simulink model "SiMappedEngine"  (R2023b)
settings: Solver=VariableStepAuto  StartTime=0.0  StopTime=inf  RelTol=1e-3  EnableMultiTasking=on
model workspace (MAT data in the model file):
  AccPwrTbl = Simulink.Parameter
  AccPwrTbl.Value = [0 0]
  AccPwrTbl.DataType = 'double'
  AccPwrTbl.Complexity = 'real'
  AccPwrTbl.Dimensions = [1 2]
  AccSpdBpts = Simulink.Parameter
  AccSpdBpts.Value = [300 750]
  AccSpdBpts.DataType = 'double'
  AccSpdBpts.Complexity = 'real'
  AccSpdBpts.Dimensions = [1 2]
  AfrStoich = Simulink.Parameter
  AfrStoich.Value = 14.6
  AfrStoich.DataType = 'double'
  AfrStoich.Complexity = 'real'
  AfrStoich.Dimensions = [1 1]
  Cps = Simulink.Parameter
  Cps.Value = 2
  Cps.DataType = 'double'
  Cps.Complexity = 'real'
  Cps.Dimensions = [1 1]
  NCyl = Simulink.Parameter
  NCyl.Value = 4
  NCyl.DataType = 'double'
  NCyl.Complexity = 'real'
  NCyl.Dimensions = [1 1]
  Pstd = Simulink.Parameter
  Pstd.Value = 101325
  Pstd.DataType = 'double'
  Pstd.Complexity = 'real'
  Pstd.Dimensions = [1 1]
  Rair = Simulink.Parameter
  Rair.Value = 287
  Rair.DataType = 'double'
  Rair.Complexity = 'real'
  Rair.Dimensions = [1 1]
  TimeCnstECP = Simulink.Parameter
  TimeCnstECP.Value = 0.125
  TimeCnstECP.DataType = 'double'
  TimeCnstECP.Complexity = 'real'
  TimeCnstECP.Dimensions = [1 1]
  TimeCnstEGR = Simulink.Parameter
  TimeCnstEGR.Value = 0.125
  TimeCnstEGR.DataType = 'double'
  TimeCnstEGR.Complexity = 'real'
  TimeCnstEGR.Dimensions = [1 1]
  TimeCnstETC = Simulink.Parameter
  TimeCnstETC.Value = 0.085
  TimeCnstETC.DataType = 'double'
  TimeCnstETC.Complexity = 'real'
  TimeCnstETC.Dimensions = [1 1]
  TimeCnstICP = Simulink.Parameter
  TimeCnstICP.Value = 0.125
  TimeCnstICP.DataType = 'double'
  TimeCnstICP.Complexity = 'real'
  TimeCnstICP.Dimensions = [1 1]
  TimeCnstIVL = Simulink.Parameter
  TimeCnstIVL.Value = 0.125
  TimeCnstIVL.DataType = 'double'
  TimeCnstIVL.Complexity = 'real'
  TimeCnstIVL.Dimensions = [1 1]
  TimeCnstMFA = Simulink.Parameter
  TimeCnstMFA.Value = 0.125
  TimeCnstMFA.DataType = 'double'
  TimeCnstMFA.Complexity = 'real'
  TimeCnstMFA.Dimensions = [1 1]
  TimeCnstSWVA = Simulink.Parameter
  TimeCnstSWVA.Value = 0.125
  TimeCnstSWVA.DataType = 'double'
  TimeCnstSWVA.Complexity = 'real'
  TimeCnstSWVA.Dimensions = [1 1]
  TimeCnstVCR = Simulink.Parameter
  TimeCnstVCR.Value = 0.125
  TimeCnstVCR.DataType = 'double'
  TimeCnstVCR.Complexity = 'real'
  TimeCnstVCR.Dimensions = [1 1]
  TimeCnstVGT = Simulink.Parameter
  TimeCnstVGT.Value = 0.15
  TimeCnstVGT.DataType = 'double'
  TimeCnstVGT.Complexity = 'real'
  TimeCnstVGT.Dimensions = [1 1]
  TimeCnstVIRL = Simulink.Parameter
  TimeCnstVIRL.Value = 0.125
  TimeCnstVIRL.DataType = 'double'
  TimeCnstVIRL.Complexity = 'real'
  TimeCnstVIRL.Dimensions = [1 1]
  TimeCnstWGA = Simulink.Parameter
  TimeCnstWGA.Value = 0.15
  TimeCnstWGA.DataType = 'double'
  TimeCnstWGA.Complexity = 'real'
  TimeCnstWGA.Dimensions = [1 1]
  Tstd = Simulink.Parameter
  Tstd.Value = 293.15
  Tstd.DataType = 'double'
  Tstd.Complexity = 'real'
  Tstd.Dimensions = [1 1]
  Vd = Simulink.Parameter
  Vd.Value = 0.0015
  Vd.DataType = 'double'
  Vd.Complexity = 'real'
  Vd.Dimensions = [1 1]
  f_air = Simulink.Parameter
  f_air.Value = [0 0 0 0 0 0 0 0 0 0 0 0 ... (256 elements, 16x16)]
  f_air.DataType = 'double'
  f_air.Complexity = 'real'
  f_air.Dimensions = [16 16]
  f_air_3d = Simulink.Parameter
  f_air_3d.Value = [0 0 0 0 0 0 0 0 0 0 0 0 ... (768 elements, 16x16x3)]
  f_air_3d.DataType = 'double'
  f_air_3d.Complexity = 'real'
  f_air_3d.Dimensions = [16 16 3]
  f_co = Simulink.Parameter
  f_co.Value = [0 0 0 0 0 0 0 0 0 0 0 0 ... (256 elements, 16x16)]
  f_co.DataType = 'double'
  f_co.Complexity = 'real'
  f_co.Dimensions = [16 16]
  f_co2 = Simulink.Parameter
  f_co2.Value = [0 0 0 0 0 0 0 0 0 0 0 0 ... (256 elements, 16x16)]
  f_co2.DataType = 'double'
  f_co2.Complexity = 'real'
  f_co2.Dimensions = [16 16]
  f_co2_3d = Simulink.Parameter
  f_co2_3d.Value = [0 0 0 0 0 0 0 0 0 0 0 0 ... (768 elements, 16x16x3)]
  f_co2_3d.DataType = 'double'
  f_co2_3d.Complexity = 'real'
  f_co2_3d.Dimensions = [16 16 3]
  f_co_3d = Simulink.Parameter
  f_co_3d.Value = [0 0 0 0 0 0 0 0 0 0 0 0 ... (768 elements, 16x16x3)]
  f_co_3d.DataType = 'double'
  f_co_3d.Complexity = 'real'
  f_co_3d.Dimensions = [16 16 3]
  f_eff = Simulink.Parameter
  f_eff.Value = [0 500 371.271960128 330.481212278 314.18997588 303.929242619 293.064446496 287.965450467 287.965450467 287.965450467 287.965450467 287.965450467 ... (256 elements, 16x16)]
  f_eff.DataType = 'double'
  f_eff.Complexity = 'real'
  f_eff.Dimensions = [16 16]
  f_eff_3d = Simulink.Parameter
  f_eff_3d.Value = [0 525 525 525 525 525 525 525 525 525 525 525 ... (768 elements, 16x16x3)]
  f_eff_3d.DataType = 'double'
  f_eff_3d.Complexity = 'real'
  f_eff_3d.Dimensions = [16 16 3]
  f_fuel = Simulink.Parameter
  f_fuel.Value = [0 0 0 0 0 0 0 0 0 0 0 0 ... (256 elements, 16x16)]
  f_fuel.DataType = 'double'
  f_fuel.Complexity = 'real'
  f_fuel.Dimensions = [16 16]
  f_fuel_3d = Simulink.Parameter
  f_fuel_3d.Value = [0 0 0 0 0 0 0 0 0 0 0 0 ... (768 elements, 16x16x3)]
  f_fuel_3d.DataType = 'double'
  f_fuel_3d.Complexity = 'real'
  f_fuel_3d.Dimensions = [16 16 3]
  f_hc = Simulink.Parameter
  f_hc.Value = [0 0 0 0 0 0 0 0 0 0 0 0 ... (256 elements, 16x16)]
  f_hc.DataType = 'double'
  f_hc.Complexity = 'real'
  f_hc.Dimensions = [16 16]
  f_hc_3d = Simulink.Parameter
  f_hc_3d.Value = [0 0 0 0 0 0 0 0 0 0 0 0 ... (768 elements, 16x16x3)]
  f_hc_3d.DataType = 'double'
  f_hc_3d.Complexity = 'real'
  f_hc_3d.Dimensions = [16 16 3]
  f_nox = Simulink.Parameter
  f_nox.Value = [0 0 0 0 0 0 0 0 0 0 0 0 ... (256 elements, 16x16)]
  f_nox.DataType = 'double'
  f_nox.Complexity = 'real'
  f_nox.Dimensions = [16 16]
  f_nox_3d = Simulink.Parameter
  f_nox_3d.Value = [0 0 0 0 0 0 0 0 0 0 0 0 ... (768 elements, 16x16x3)]
  f_nox_3d.DataType = 'double'
  f_nox_3d.Complexity = 'real'
  f_nox_3d.Dimensions = [16 16 3]
  f_pm = Simulink.Parameter
  f_pm.Value = [0  0  0  0  0  0  0  0  0  0  0  0  0  0  0  0; 0  0  0  0  0  0  0  0  0  0  0  0  0  0  0  0; 0  0  0  0  0  0  0  0  0  0  0  0  0  0  0  0; 0  0  0  0  0  0  0  0  0  0  0  0  0  0  0  0; 0  0  0  0  0  0  0  0  0  0  0  0  0  0  0  0; 0  0  0  0  0  0  0  0  0  0  0  0  0  0  0  0; 0  0  0  0  0  0  0  0  0  0  0  0  0  0  0  0; 0  0  0  0  0  0  0  0  0  0  0  0  0  0  0  0; 0  0  0  0  0  0  0  0  0  0  0  0  0  0  0  0; 0  0  0  0  0  0  0  0  0  0  0  0  0  0  0  0; 0  0  0  0  0  0  0  0  0  0  0  0  0  0  0  0; 0  0  0  0  0  0  0  0  0  0  0  0  0  0  0  0; 0  0  0  0  0  0  0  0  0  0  0  0  0  0  0  0; 0  0  0  0  0  0  0  0  0  0  0  0  0  0  0  0; 0  0  0  0  0  0  0  0  0  0  0  0  0  0  0  0; 0  0  0  0  0  0  0  0  0  0  0  0  0  0  0  0]
  f_pm.DataType = 'double'
  f_pm.Complexity = 'real'
  f_pm.Dimensions = [16 16]
  f_pm_3d = Simulink.Parameter
  f_pm_3d.Value = reshape([0 0 0 0 0 0 0 0 0 0 0 0 0 0 0 0 0 0 0 0 0 0 0 0 0 0 0 0 0 0 0 0 0 0 0 0 0 0 0 0 0 0 0 0 0 0 0 0 0 0 0 0 0 0 0 0 0 0 0 0 0 0 0 0 0 0 0 0 0 0 0 0 0 0 0 0 0 0 0 0 0 0 0 0 0 0 0 0 0 0 0 0 0 0 0 0 0 0 0 0 0 0 0 0 0 0 0 0 0 0 0 0 0 0 0 0 0 0 0 0 0 0 0 0 0 0 0 0 0 0 0 0 0 0 0 0 0 0 0 0 0 0 0 0 0 0 0 0 0 0 0 0 0 0 0 0 0 0 0 0 0 0 0 0 0 0 0 0 0 0 0 0 0 0 0 0 0 0 0 0 0 0 0 0 0 0 0 0 0 0 0 0 0 0 0 0 0 0 0 0 0 0 0 0 0 0 0 0 0 0 0 0 0 0 0 0 0 0 0 0 0 0 0 0 0 0 0 0 0 0 0 0 0 0 0 0 0 0 0 0 0 0 0 0 0 0 0 0 0 0 0 0 0 0 0 0 0 0 0 0 0 0 0 0 0 0 0 0 0 0 0 0 0 0 0 0 0 0 0 0 0 0 0 0 0 0 0 0 0 0 0 0 0 0 0 0 0 0 0 0 0 0 0 0 0 0 0 0 0 0 0 0 0 0 0 0 0 0 0 0 0 0 0 0 0 0 0 0 0 0 0 0 0 0 0 0 0 0 0 0 0 0 0 0 0 0 0 0 0 0 0 0 0 0 0 0 0 0 0 0 0 0 0 0 0 0 0 0 0 0 0 0 0 0 0 0 0 0 0 0 0 0 0 0 0 0 0 0 0 0 0 0 0 0 0 0 0 0 0 0 0 0 0 0 0 0 0 0 0 0 0 0 0 0 0 0 0 0 0 0 0 0 0 0 0 0 0 0 0 0 0 0 0 0 0 0 0 0 0 0 0 0 0 0 0 0 0 0 0 0 0 0 0 0 0 0 0 0 0 0 0 0 0 0 0 0 0 0 0 0 0 0 0 0 0 0 0 0 0 0 0 0 0 0 0 0 0 0 0 0 0 0 0 0 0 0 0 0 0 0 0 0 0 0 0 0 0 0 0 0 0 0 0 0 0 0 0 0 0 0 0 0 0 0 0 0 0 0 0 0 0 0 0 0 0 0 0 0 0 0 0 0 0 0 0 0 0 0 0 0 0 0 0 0 0 0 0 0 0 0 0 0 0 0 0 0 0 0 0 0 0 0 0 0 0 0 0 0 0 0 0 0 0 0 0 0 0 0 0 0 0 0 0 0 0 0 0 0 0 0 0 0 0 0 0 0 0 0 0 0 0 0 0 0 0 0 0 0 0 0 0 0 0 0 0 0 0 0 0 0 0 0 0 0 0 0 0 0 0 0 0 0 0 0 0 0 0 0 0 0 0 0 0 0 0 0 0 0 0 0 0 0 0 0 0 0 0 0 0 0 0 0 0 0 0 0 0 0 0 0 0 0 0 0 0 0 0 0 0 0 0 0 0 0 0 0 0 0 0 0 0 0 0 0 0 0 0 0 0 0 0 0 0 0 0 0 0 0 0 0 0 0 0 0 0 0 0 0 0 0 0 0 0 0 0 0 0 0 0 0 0 0 0 0 0 0 0 0 0 0 0 0 0 0 0 0 0 0 0 0 0 0 0 0 0 0 0 0], [16 16 3])
  f_pm_3d.DataType = 'double'
  f_pm_3d.Complexity = 'real'
  f_pm_3d.Dimensions = [16 16 3]
  f_tbrake = Simulink.Parameter
  f_tbrake.Value = [0 15 26.4285714286 37.8571428571 49.2857142857 60.7142857143 72.1428571429 75.6797764808 75.6797764808 75.6797764808 75.6797764808 75.6797764808 ... (256 elements, 16x16)]
  f_tbrake.DataType = 'double'
  f_tbrake.Complexity = 'real'
  f_tbrake.Dimensions = [16 16]
  f_tbrake_3d = Simulink.Parameter
  f_tbrake_3d.Value = [0 14.25 14.25 14.25 14.25 14.25 14.25 14.25 14.25 14.25 14.25 14.25 ... (768 elements, 16x16x3)]
  f_tbrake_3d.DataType = 'double'
  f_tbrake_3d.Complexity = 'real'
  f_tbrake_3d.Dimensions = [16 16 3]
  f_tbrake_engtmp_bpt = Simulink.Parameter
  f_tbrake_engtmp_bpt.Value = [233.15 273.15 373.15]
  f_tbrake_engtmp_bpt.DataType = 'double'
  f_tbrake_engtmp_bpt.Complexity = 'real'
  f_tbrake_engtmp_bpt.Dimensions = [1 3]
  f_tbrake_n_bpt = Simulink.Parameter
  f_tbrake_n_bpt.Value = [0 750 1053.57142857 1357.14285714 1660.71428571 1964.28571429 2267.85714286 2571.42857143 2875 3178.57142857 3482.14285714 3785.71428571 4089.28571429 4392.85714286 4696.42857143 5000]
  f_tbrake_n_bpt.DataType = 'double'
  f_tbrake_n_bpt.Complexity = 'real'
  f_tbrake_n_bpt.Dimensions = [1 16]
  f_tbrake_t_bpt = Simulink.Parameter
  f_tbrake_t_bpt.Value = [0 15 26.4285714286 37.8571428571 49.2857142857 60.7142857143 72.1428571429 83.5714285714 95 106.428571429 117.857142857 129.285714286 140.714285714 152.142857143 163.571428571 175]
  f_tbrake_t_bpt.DataType = 'double'
  f_tbrake_t_bpt.Complexity = 'real'
  f_tbrake_t_bpt.Dimensions = [1 16]
  f_texh = Simulink.Parameter
  f_texh.Value = [730.342454351 730.703124121 753.727232127 774.716518351 790.943395964 828.546144893 892.868946573 904.250339899 904.250339899 904.250339899 904.250339899 904.250339899 ... (256 elements, 16x16)]
  f_texh.DataType = 'double'
  f_texh.Complexity = 'real'
  f_texh.Dimensions = [16 16]
  f_texh_3d = Simulink.Parameter
  f_texh_3d.Value = [693.825331629 694.167967914 694.167967914 694.167967914 694.167967914 694.167967914 694.167967914 694.167967914 694.167967914 694.167967914 694.167967914 694.167967914 ... (768 elements, 16x16x3)]
  f_texh_3d.DataType = 'double'
  f_texh_3d.Complexity = 'real'
  f_texh_3d.Dimensions = [16 16 3]
  f_twc_eff_co = Simulink.Parameter
  f_twc_eff_co.Value = [0.17 0.25 0.45 0.99 0.99 0.99 0.99]
  f_twc_eff_co.DataType = 'double'
  f_twc_eff_co.Complexity = 'real'
  f_twc_eff_co.Dimensions = [1 7]
  f_twc_eff_hc = Simulink.Parameter
  f_twc_eff_hc.Value = [0.21 0.375 0.75 0.98 0.98 0.98 0.98]
  f_twc_eff_hc.DataType = 'double'
  f_twc_eff_hc.Complexity = 'real'
  f_twc_eff_hc.Dimensions = [1 7]
  f_twc_eff_lam = Simulink.Parameter
  f_twc_eff_lam.Value = [0.909090909 0.944055944 0.979020979 1 1.013986014 1.048951049 1.083916084]
  f_twc_eff_lam.DataType = 'double'
  f_twc_eff_lam.Complexity = 'real'
  f_twc_eff_lam.Dimensions = [1 7]
  f_twc_eff_nox = Simulink.Parameter
  f_twc_eff_nox.Value = [0.98 0.98 0.98 0.97 0.05 0.02 0]
  f_twc_eff_nox.DataType = 'double'
  f_twc_eff_nox.Complexity = 'real'
  f_twc_eff_nox.Dimensions = [1 7]
libraries: autolibhevctrlrcommon x1, autolibpowerinfoutils x1, autolibsharedmappedengines x1, autolibutils x1
(part 1 of 2)
settings Model: DataDictionary=SiMappedEngine.sldd  ModifiedByFormat=The MathWorks, Inc.  Creator=The MathWorks, Inc.  LastModifiedBy=The MathWorks, Inc.
settings SolverCC: AlgebraicLoopSolver=TrustRegion  DecoupledContinuousIntegration=on  MaxZcPerStep=1
settings DataIOCC: DSMLogging=off  ReturnWorkspaceOutputs=off
settings DebuggingCC: UnconnectedInputMsg=warning  UnconnectedOutputMsg=warning  UnconnectedLineMsg=warning  SubsystemReferenceDiagnosticForUnitTest=warning  ArithmeticOperatorsInVariantConditions=warning
settings ModelReferenceCC: EnableRefExpFcnMdlSchedulingChecks=on
settings SFSimCC: SimUseLocalCustomCode=off  CustomCodeUndefinedFunction=UseInterfaceOnly
settings RTWCC: RTWUseLocalCustomCode=off  DLArmComputeVersion=19.05
settings CodeAppCC: StateflowObjectComments=on
settings GRTTargetCC: TargetLangStandard=C89/C90 (ANSI)
settings ConfigComp: CovMetricSettings=dsw  CovSaveCumulativeToWorkspaceVar=on  CovSaveSingleToWorkspaceVar=on  CovExternalEMLEnable=off
settings SimscapeCC: SimscapeNormalizeSystem=off  SimscapeNominalValues={1, 'bar'; 1, 'cm^3/s'; 1, 'bar*kg/s'; 1, 'kJ/kg'; 1, 'kW'}

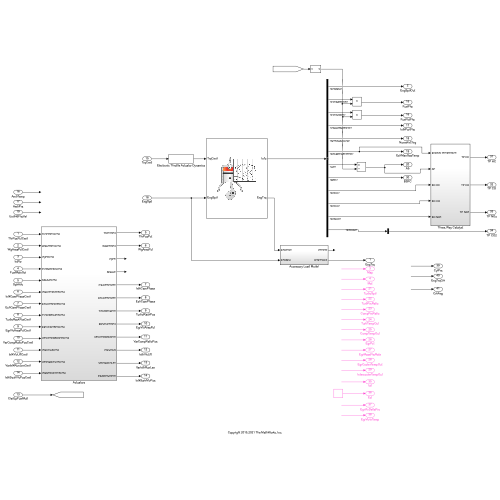
[thumbnail: Simulink's stored preview of the top-level diagram]
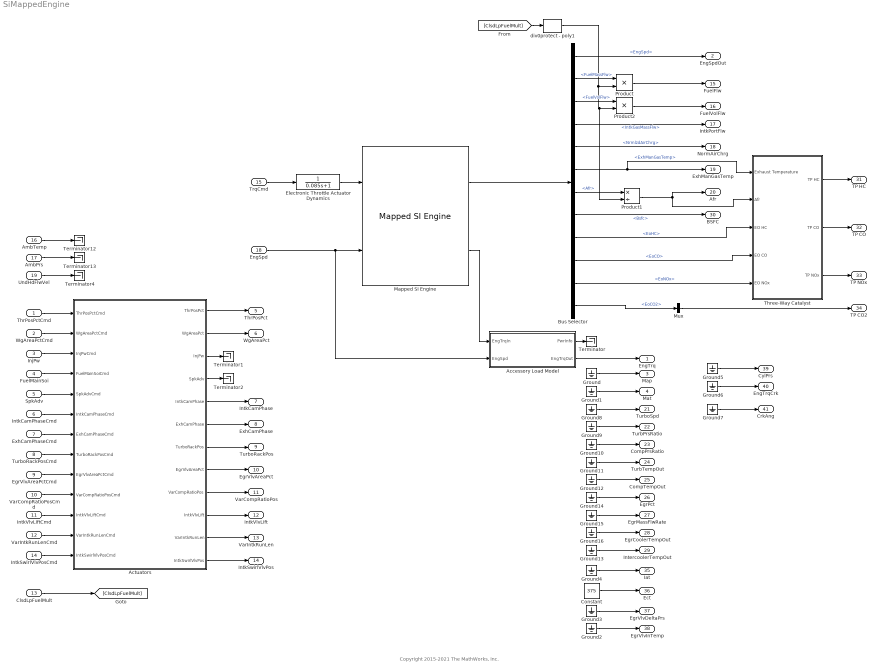
== system SiMappedEngine ==
  note: Copyright 2015-2021 The MathWorks, Inc.
  ThrPosPctCmd : Inport
  WgAreaPctCmd : Inport  Port=2
  InjPw : Inport  Port=3
  FuelMainSoi : Inport  Port=4
  SpkAdv : Inport  Port=5
  IntkCamPhaseCmd : Inport  Port=6
  ExhCamPhaseCmd : Inport  Port=7
  TurboRackPosCmd : Inport  Port=8
  EgrVlvAreaPctCmd : Inport  Port=9
  VarCompRatioPosCmd : Inport  Port=10
  IntkVlvLiftCmd : Inport  Port=11
  VarIntkRunLenCmd : Inport  Port=12
  ClsdLpFuelMult : Inport  Port=13  Unit=1
  IntkSwirlVlvPosCmd : Inport  Port=14
  TrqCmd : Inport  Port=15  Unit=N*m
  AmbTemp : Inport  Port=16  Unit=K
  AmbPrs : Inport  Port=17  Unit=Pa
  EngSpd : Inport  Port=18  Interpolate=off
  UndHdFlwVel : Inport  Port=19  Unit=m/s
  Accessory Load Model : Subsystem
  Actuators : Subsystem
  Bus Selector : BusSelector  OutputSignals=EngSpd,FuelMassFlw,FuelVolFlw,IntkGasMassFlw,NrmlzdAirChrg,ExhManGasTemp,Afr,Bsfc,EoHC,EoCO,EoNOx,EoCO2
  Constant : Constant  Value=375
  Electronic Throttle Actuator Dynamics : TransferFcn  Denominator=[0.085 1]
  Ground{,1..16} (17 alike) : Ground
  Mapped SI Engine : autolibsharedmappedengines/Mapped SI Engine  TurboLagCheckbox=off  EngTmpInpEnbl=off  rowVarName=TrqCmd  f_tbrake_t_bpt=f_tbrake_t_bpt  colVarName=EngSpd  f_tbrake_n_bpt=f_tbrake_n_bpt  f_tbrake_engtmp_bpt=f_tbrake_engtmp_bpt  NCyl=NCyl  Cps=Cps  Vd=Vd  Lhv=46e6  Sg=0.745  Rair=Rair  Pstd=Pstd  Tstd=Tstd  Use1=on  Use2=on  Use3=on  Use4=on  Use5=on  Use6=on  Use7=on  Use8=on  Use9=on  Use10=off  f_tbrake_bst=[0, 79.51 81.38 91.45 97.78 102.6 106.2 109.6 111.6 113.4 113.9 113.3 115 111.9 108.1 105]  tau_thr=0.2  tau_bst_rising=1.5  tau_bst_falling=1  tq_blend_frac=0.01  Name1=Brake Torque  f_tbrake=f_tbrake  f_tbrake_3d=cat(3,[0,-13.6738264268725,-14.7516162546659,-15.6514273193086,-16.3079930289672,-16.8655148686042,-17.3519404917215,-18.0021012886426,-18.8938299980449,-19.7110729335300,-20.4110131019604,-20.8892101554636,-21.3889975517772,-22.0965449137417,-22.8606364021968,-23.5713693096665;15.0034460820826,15.0034460820826,15.0085465602505,15.0543856756029,15.0236112005788,14.9329468853953,15.0994373826734,15.0083764795969,14.9491141032579,14.9727796153047,14.9824150502786,15.0208742146344,14.5655072782863,14.9611058168861,15.0796566994499,15.0002658789506;26.4289521304740,26.4289521304740,26.4289139604196,26.4408235747463,26.5407413158044,26.4802770030823,26.5299269544112,26.4321714966371,26.3084102264475,26.4325791487006,26.4236524787126,26.5965994622732,26.3199729302878,26.4983579045646,26.4364346449783,26.4287308294291;37.8539339756192,37.8539339756192,37.8525565353244,37.8378458922433,37.9209957202538,37.8696500366897,37.8568037097691,37.9028487613723,37.8451441941685,37.7078129749522,37.9340133199123,37.8121210964161,37.9346007179415,37.8789400100985,37.7978559494457,37.8571176403673;49.2854604963563,49.2854604963563,49.2989783920396,49.2919407086180,49.2849294911958,49.2696605805777,49.2820498979492,49.2727728646495,49.2902474719513,49.2601580879798,49.2322295400638,49.2852362217095,49.2893776657938,49.2596979604933,49.4127743785610,49.2857954882698;60.7146317399387,60.7146317399387,60.7355154506901,60.7239172372991,60.7217710948102,60.7137324397883,60.7143874707284,60.7062997394405,60.7052144430060,60.7126110381044,60.5907223881537,60.6208027350816,60.6952855278890,60.8471808967815,60.7703327333014,60.7141065945303;72.0173711594535,72.0173711594535,72.1458656317514,72.1313569896252,72.1526641458003,72.1379273224849,72.1394015443471,72.1463163027315,72.1691439257264,72.2315917404871,72.1046693089443,72.1951353754188,72.1155687058044,72.2288384599957,72.1363768844456,72.1428649823425;77.7345012802114,77.7345012802114,84.5839183476413,83.6470935593627,83.5827407998509,83.5795940255237,83.5969146489249,83.5154963867684,83.5229988861936,83.5616009871909,83.6888627929518,83.6772286993939,83.7474008585288,83.6230781067179,83.5070071419442,83.5722038905255;77.7345012802114,77.7345012802114,95.0523640290054,94.6478360873227,94.9574888217504,95.1522514962210,94.9257361523427,94.9801883923262,94.9895081579654,95.1070597041224,95.0076760091942,95.0431472512251,95.1405880340105,94.8695895431046,94.9704933892662,95.0003976667408;77.7345012802114,77.7345012802114,101.987276870835,106.720510143102,107.434212780557,104.902851113535,106.376450721902,106.404252185671,106.509764410733,106.374561907885,106.406074819820,106.378193853297,106.468588227905,106.711986977064,106.488166811887,106.429122510611;77.7345012802114,77.7345012802114,102.207184311641,117.967350541924,117.595066388461,117.934473027129,117.808663275139,117.881260178262,117.941786510634,117.876160181786,117.923000258289,117.724496544638,117.865430922165,117.891943502543,117.622108822166,117.739296920672;77.7345012802114,77.7345012802114,102.207184311641,120.914696442157,129.348729885173,129.449253984265,129.212966694762,129.363648158656,129.205714699780,129.138906124197,129.276684278753,129.500764139179,128.733663374355,129.139204799969,129.345410933638,129.187085301851;77.7345012802114,77.7345012802114,102.207184311641,120.914696442157,132.039529042327,140.413809507162,140.916381925873,140.709390494329,140.970209272488,140.670221267529,140.572232588817,140.837355250507,140.591631198379,140.735297072228,140.719702448301,140.693844078338;77.7345012802114,77.7345012802114,102.207184311641,120.914696442157,132.039529042327,143.890412333636,150.134747173048,152.352748266079,150.528590427068,152.375101731327,151.601271491801,152.024935398035,152.224075104129,151.651055675596,151.234127013963,151.956564108969;77.7345012802114,77.7345012802114,102.207184311641,120.914696442157,132.039529042327,143.890412333636,150.134747173048,155.406512101229,150.528590427068,158.598225904784,163.027088204109 ...(+9065 chars)])  Name2=Air Mass Flow  f_air=f_air  f_air_3d=cat(3,[0,0,0,0,0,0,0,0,0,0,0,0,0,0,0,0;0,0.00243798018228422,0.00314861633804768,0.00402773022646749,0.00490679644301041,0.00584129203751529,0.00679621076249438,0.00775996419325510,0.00876445595078949,0.00981835158328834,0.0109384385877509,0.0119575142240558,0.0131074751940218,0.0145956507047312,0.0159715846162714,0.0172963402153914;0,0.00311127166114377,0.00425400462966738,0.00539186788588643,0.00651952607432526,0.00776541678457505,0.00898354755753331,0.0102260491477933,0.0115139948349982,0.0127849865807937,0.0141406918306152,0.0155106804204685,0.0169635764523402,0.0185836755533759,0.0202250226010108,0.0218743169255529;0,0.00390992759617313,0.00532019173726916,0.00675428305659032,0.00814776118783315,0.00968297088566079,0.0111876342865897,0.0126943288849878,0.0142809635791296,0.0157972134201687,0.0174880936115939,0.0191202643005044,0.0207902378156622,0.0226424070337401,0.0245798171274491,0.0265200962769632;0,0.00471248335909574,0.00641581369137303,0.00812916559944056,0.00987469203316234,0.0116439463515056,0.0134160929079301,0.0151710754125667,0.0168764807857917,0.0187598804008532,0.0208140773825812,0.0226567027825258,0.0246386628679306,0.0267774515252309,0.0289907690311517,0.0312298756288423;0,0.00554390955043716,0.00751426225777199,0.00949918913692272,0.0115035444104902,0.0134674691075210,0.0155056255831980,0.0175070593032372,0.0196241231433751,0.0217999811216041,0.0241277473887585,0.0262211348582284,0.0285555800226685,0.0309600153601999,0.0334771886663496,0.0360503618807771;0,0.00661166990661863,0.00863640554377020,0.0108963363534636,0.0131582178749028,0.0153584375796297,0.0176531994041711,0.0200120001601262,0.0224205546243444,0.0249730016255865,0.0272866528982126,0.0298181210005599,0.0324396741914578,0.0351875844807284,0.0380167927386357,0.0409465645960739;0,0.00709048856805421,0.0100138368138258,0.0122815333609596,0.0148738141752333,0.0173389077943237,0.0199095004145845,0.0226862036827974,0.0252829294100960,0.0278466508867810,0.0305804147512288,0.0334314552875712,0.0363917787051532,0.0394199960939184,0.0426609250609142,0.0455975299745196;0,0.00709048856805421,0.0112830160693863,0.0137682602137922,0.0164633051957177,0.0193879632136123,0.0222294826817616,0.0249933836167389,0.0279025734510493,0.0309012412590225,0.0339880300500983,0.0371276954178573,0.0403582824246840,0.0439330938492141,0.0471871081556525,0.0507467821663682;0,0.00709048856805421,0.0125196458234850,0.0153292830264171,0.0178500303127613,0.0200085042006289,0.0243022038405892,0.0274707135977572,0.0307221743749666,0.0340396004161378,0.0373661470278661,0.0408745895262397,0.0444828751872244,0.0482734578668554,0.0519172033398123,0.0555537972752765;0,0.00709048856805421,0.0125506479073243,0.0182084301352740,0.0202840690475063,0.0232146905454237,0.0266355569688144,0.0300794178139807,0.0336013300832806,0.0372418755581227,0.0409239031329721,0.0446977424880355,0.0486785225558507,0.0527474098019116,0.0566549478235795,0.0606006482947292;0,0.00709048856805421,0.0125506479073243,0.0190885348022137,0.0237943506792112,0.0258904380043180,0.0291503102749100,0.0328420004322395,0.0367796984931652,0.0406484132996543,0.0447214150295748,0.0489556099830268,0.0530937300953106,0.0576792545106145,0.0619573984770550,0.0664052497978025;0,0.00709048856805421,0.0125506479073243,0.0190885348022137,0.0258485107458050,0.0303966301597821,0.0322495965396904,0.0358908672679084,0.0400152633948443,0.0441810034694858,0.0487138474593659,0.0531417035706776,0.0578582817822865,0.0626003505069147,0.0667896107223227,0.0717917339663930;0,0.00709048856805421,0.0125506479073243,0.0190885348022137,0.0258485107458050,0.0336945949729501,0.0420088397544187,0.0398412172140341,0.0493355546428196,0.0477724454535298,0.0525028674556899,0.0571750062515294,0.0620065991325053,0.0668445480192095,0.0731803581820234,0.0788759717452155;0,0.00709048856805421,0.0125506479073243,0.0190885348022137,0.0258485107458050,0.0336945949729501,0.0420088397544187,0.0475964679450510,0.0493355546428196,0.0551550926188752,0.0609972993183876 ...(+9137 chars)])  Name3=Fuel Flow  f_fuel=f_fuel  f_fuel_3d=cat(3,[0,0,0,0,0,0,0,0,0,0,0,0,0,0,0,0;0,0.000166984943992070,0.000215658653290937,0.000275871933319691,0.000336081948151398,0.000400088495720226,0.000465493887842081,0.000531504396798294,0.000600305202108869,0.000672489834471804,0.000749208122448694,0.000819007823565468,0.000897772273563136,0.000999702103063781,0.00109394415179941,0.00118468083667064;0,0.000213100798708477,0.000291370180114204,0.000369306019581262,0.000446542881803100,0.000531877861957196,0.000615311476543377,0.000700414325191323,0.000788629783219051,0.000875684012383128,0.000968540536343508,0.00106237537126496,0.00116188879810549,0.00127285448995726,0.00138527552061718,0.00149824088531184;0,0.000267803260011858,0.000364396694333504,0.000462622127163720,0.000558065834783092,0.000663217183949369,0.000766276320999294,0.000869474581163547,0.000978148190351341,0.00108200091918964,0.00119781463093109,0.00130960714387017,0.00142398889148371,0.00155084979683151,0.00168354911831843,0.00181644495047693;0,0.000322772832814776,0.000439439293929660,0.000556792164345244,0.000676348769394681,0.000797530572020931,0.000918910473145896,0.00103911475428539,0.00115592334149258,0.00128492331512693,0.00142562173853296,0.00155182895770725,0.00168757964848840,0.00183407202227609,0.00198566911172272,0.00213903257731796;0,0.000379719832221723,0.000514675497107671,0.000650629392939912,0.000787914000718505,0.000922429390926093,0.00106202914953411,0.00119911365090666,0.00134411802351884,0.00149314939189069,0.00165258543758620,0.00179596814097455,0.00195586164538826,0.00212054899727397,0.00229295812783217,0.00246920286854638;0,0.000452854103193057,0.000591534626285630,0.000746324407771482,0.000901247799650874,0.00105194777942669,0.00120912324686104,0.00137068494247440,0.00153565442632496,0.00171047956339634,0.00186894882864470,0.00204233705483287,0.00222189549256560,0.00241010852607729,0.00260388991360518,0.00280455921890917;0,0.000485649901921521,0.000685879233823688,0.000841200915134221,0.00101875439556392,0.00118759642426874,0.00136366441195784,0.00155384956731489,0.00173170749384219,0.00190730485525898,0.00209454895556362,0.00228982570462816,0.00249258758254474,0.00269999973246016,0.00292198116855577,0.00312311849140545;0,0.000485649901921521,0.000772809319820981,0.000943031521492620,0.00112762364354231,0.00132794268586385,0.00152256730696998,0.00171187559018760,0.00191113516788009,0.00211652337390565,0.00232794726370537,0.00254299283683954,0.00276426591949890,0.00300911601706946,0.00323199370929127,0.00347580699769645;0,0.000485649901921521,0.000857509987909935,0.00104995089222035,0.00122260481594255,0.00137044549319376,0.00166453450962940,0.00188155572587378,0.00210425851883333,0.00233147948055739,0.00255932513889494,0.00279962941960546,0.00304677227309756,0.00330640122375722,0.00355597283149399,0.00380505460789565;0,0.000485649901921521,0.000859633418309883,0.00124715274899137,0.00138931979777440,0.00159004729763176,0.00182435321704208,0.00206023409684800,0.00230146096460826,0.00255081339439197,0.00280300706390220,0.00306148921150928,0.00333414538053772,0.00361283628780216,0.00388047587832737,0.00415072933525542;0,0.000485649901921521,0.000859633418309883,0.00130743389056258,0.00162975004652132,0.00177331767152863,0.00199659659417191,0.00224945208439997,0.00251915743103871,0.00278413789723660,0.00306311061846403,0.00335312397144019,0.00363655685584319,0.00395063387059003,0.00424365742993527,0.00455741961991122;0,0.000485649901921521,0.000859633418309883,0.00130743389056258,0.00189555239988597,0.00208196096984809,0.00220887647532126,0.00245827857999372,0.00274077146540030,0.00302609612804698,0.00334325139727166,0.00363984271032038,0.00396289601248538,0.00428769524019964,0.00458379846832863,0.00520894285221681;0,0.000485649901921521,0.000859633418309883,0.00130743389056258,0.00189555239988597,0.00259892902111487,0.00340108485980915,0.00272885049411192,0.00411088513172180,0.00340842219274614,0.00385020001288389,0.00398787812484512,0.00433370136514574,0.00469097715158387 ...(+9908 chars)])  Name4=Exhaust Temperature  f_texh=f_texh  f_texh_3d=cat(3,[737.907113763617,737.907113763617,696.820165367239,774.049075818828,840.786359554579,903.838236096434,967.200910655749,1002.74075874828,1012.71729177990,1031.94000420684,1064.78457862769,1067.29521471648,1071.89247123133,1106.91922705762,1124.41819784223,1139.44782816948;737.907113763617,737.907113763617,696.820165367239,774.049075818828,840.786359554579,903.838236096434,967.200910655749,1002.74075874828,1012.71729177990,1031.94000420684,1064.78457862769,1067.29521471648,1071.89247123133,1106.91922705762,1124.41819784223,1139.44782816948;755.082208112884,755.082208112884,823.297755777469,881.221034181030,934.210964047041,963.419294279027,987.007225051922,1016.82903399991,1000.24965285330,1013.32659225923,1036.16284115240,1052.57236702455,1076.49835901210,1110.98959218276,1128.45097840633,1144.42264679139;772.037002214033,772.037002214033,875.875746866932,922.707853406823,945.218671089386,964.054629014275,993.591387093673,1003.65317726610,996.024264792699,1017.74780803692,1033.23344245175,1063.40453655061,1094.16141010298,1109.79033100368,1128.37869571910,1135.98640791982;793.402168165624,793.402168165624,879.301190663428,924.860724240834,952.674293644717,968.618515544313,984.911460269000,995.978176214796,974.123631131658,993.874811186928,1040.56112506944,1068.39988354457,1093.80509694083,1106.66756341525,1120.07286383497,1130.47656928185;791.792649117823,791.792649117823,892.804287534570,934.804182927649,950.264917968478,957.944203869714,979.179173872084,983.491434982593,999.025935482248,1010.76292716219,1055.27196835756,1084.28009467673,1096.06397899297,1102.06018281492,1112.69023961000,1131.05391745303;861.700075845396,861.700075845396,902.647791160960,953.786158310821,978.336272737350,988.849243805652,999.713470916476,1009.62136384468,1017.74965307258,1053.72273660870,1080.38777223473,1099.34275119018,1108.83540739255,1112.85122375699,1112.94782080380,1123.84611974638;917.462752105090,917.462752105090,928.924823204072,954.858526705702,997.430947365226,1012.09045999535,1022.19379449664,1039.25328881161,1057.78765849458,1083.71356338622,1096.67341285066,1115.70821472062,1126.82299238222,1126.59623299889,1114.30710751197,1117.21260012813;917.462752105090,917.462752105090,1038.81975747386,974.962699761948,1008.20813290058,1030.07218490084,1045.60014586410,1062.84753653739,1076.67088447148,1094.77585048953,1111.01509004292,1125.29464430527,1135.21645021122,1123.11766303610,1112.22378912667,1127.20753511812;917.462752105090,917.462752105090,1097.93084562817,1040.26624249454,1021.54429059208,1021.80900518598,1053.45470308994,1069.89208215374,1089.59478862277,1114.30266182869,1127.75479455573,1138.88672076819,1145.80722144700,1133.17254578720,1127.75920841370,1145.62106335132;917.462752105090,917.462752105090,1098.36234970405,1132.05644399615,1052.68386741604,1024.71191891219,1062.81252552398,1088.63260327452,1106.12434203191,1126.30848478453,1134.19756330860,1148.02580067901,1153.52921355718,1146.94188539490,1142.98943112126,1155.25589191691;917.462752105090,917.462752105090,1098.36234970405,1164.67992636172,1145.67743364425,1077.02800246979,1043.29697086814,1087.33531021166,1125.78926436291,1141.24992637076,1154.47114171142,1161.80517752364,1159.47096767341,1156.45987255324,1158.18292429204,1174.84699526957;917.462752105090,917.462752105090,1098.36234970405,1164.67992636172,1168.49415127559,1157.45769726052,1078.75642990539,1086.32939639484,1147.86384769643,1158.67155716235,1174.45153367655,1167.63977398731,1165.99753974412,1164.21749666157,1175.03756415226,1150.06761876987;917.462752105090,917.462752105090,1098.36234970405,1164.67992636172,1168.49415127559,1163.34799484753,1183.39262276118,1132.82956196960,1174.25455564043,1159.57945799032,1154.52008791161,1170.72995542419,1163.55685237192,1165.32941995085,1190.43765038819,1176.94579818352;917.462752105090,917.462752105090,1098.36234970405,1164.67992636172,1168.49415127559,1163.34799484753,1183.39262276118,1169.82938966886,1174.25455564043,1173.07948381242,1167.62626962956 ...(+9065 chars)])  Name5=[514.035834811904 472.420001567292 468.560027988283 467.25113080026 469.376552017678 472.466817198703 477.085817372135 482.089315297269 488.091390331625 495.511698221518 503.603605470575 513.545560314063 524.708632042863 537.901582788691 547.57773149968;372.215126833557 362.023004934345 357.061196096605 354.397690627091 353.695017513094 355.069365264177 357.083429546077 359.150328797338 361.216056662124 363.787443052002 368.052362907894 373.273609540704 379.492527390704 387.062712835118 392.829054841793;326.61409907784 316.864439849348 311.950172215081 309.623392513349 308.520317680707 308.639621388036 309.473192508284 311.206605049837 312.435624355117 314.372691523229 315.240918825382 319.20290576235 323.194337587902 328.582300779183 332.542719046893;302.302708332089 292.988583490457 288.191388571794 286.11397076702 285.309041994516 284.733243126823 284.189019193475 282.574319206257 284.12037910983 287.79556805798 288.17907837576 290.209859138972 293.679673638155 297.45343144841 300.726288347892;288.700928736811 278.551672830084 273.400833959319 270.536547804349 267.833435583205 267.119414364878 265.972950018046 266.740920363958 268.048224971445 270.838385340352 270.778373480454 272.970259132319 275.506872347887 278.72040783414 281.813869092965;284.845821006168 269.394829178651 263.982926589081 260.478586413209 257.028965789929 255.931084916756 255.874470882376 256.430426703396 258.42024291946 257.808327020541 258.950655075076 261.079050323518 263.461085730423 266.38231289239 269.295763051135;288.386442360439 264.344752526028 257.213462364171 254.168296127581 250.527881300837 249.049345022729 250.073316495023 249.665324624047 248.602086912424 249.355944667699 250.714426186754 252.515083416491 254.990022645247 258.139224389126 258.88586921331;288.386442360439 267.197275532715 251.193959608514 247.553061326459 246.301141111655 244.695607301207 242.621990784403 242.304630618562 242.866111727694 243.758994026591 244.970247326866 246.821991594926 249.775586923996 251.245282116681 253.478417008787;288.386442360439 277.668290802935 252.854894387889 243.851167532952 241.861572413297 238.689990387976 238.067198500515 238.072941982365 238.685701547209 239.312989651019 240.673403883432 242.669277941474 245.301951037108 246.789302536782 247.789414843363;288.386442360439 277.504945286633 270.702819258252 245.731480615597 238.395305310031 236.119281963407 235.324944828075 235.181758472016 235.88354482046 236.67974458838 237.758701429304 239.923633193373 242.123394230695 242.998011528535 244.273734537053;288.386442360439 277.504945286633 279.349376222353 263.18046263446 241.569205761561 235.781254475789 234.445285156959 234.881842747232 234.822376790859 235.79445272942 237.439515459863 239.43946089678 241.356663529347 242.334213324245 244.486434215002;288.386442360439 277.504945286633 279.349376222353 299.505188255346 260.338046997911 239.40420517855 235.256510952508 234.880694514868 234.31593804329 236.319225658558 237.102712721133 239.012709272806 240.75776355138 241.336977805019 256.331160738088;288.386442360439 277.504945286633 279.349376222353 299.505188255346 320.026630425816 342.9283130372 241.52452305243 328.315966517739 244.549289572305 251.858270967766 240.732881082116 242.07382019702 244.535478307747 249.496579565711 263.930188372987;288.386442360439 277.504945286633 279.349376222353 299.505188255346 320.026630425816 342.9283130372 345.883623776508 328.315966517739 317.337354078743 314.624789096503 254.725548546873 250.384805432702 271.371327381584 265.474840242786 277.521724347837;288.386442360439 277.504945286633 279.349376222353 299.505188255346 320.026630425816 342.9283130372 345.883623776508 328.315966517739 319.749039003082 318.879022253509 311.782458169383 312.350604651759 319.747883103035 320.841917879101 308.256263223954]  f_eff=f_eff  f_eff_3d=cat(3,[0,0,0,0,0,0,0,0,0,0,0,0,0,0,0,0;0,514.035834811904,472.420001567292,468.560027988283,467.251130800260,469.376552017678,472.466817198703,477.085817372135,482.089315297269,488.091390331625,495.511698221518,503.603605470575,513.545560314063,524.708632042863,537.901582788691,547.577731499680;0,372.215126833557,362.023004934345,357.061196096605,354.397690627091,353.695017513094,355.069365264177,357.083429546077,359.150328797338,361.216056662124,363.787443052002,368.052362907894,373.273609540704,379.492527390704,387.062712835118,392.829054841793;0,326.614099077840,316.864439849348,311.950172215081,309.623392513349,308.520317680707,308.639621388036,309.473192508284,311.206605049837,312.435624355117,314.372691523229,315.240918825382,319.202905762350,323.194337587902,328.582300779183,332.542719046893;0,302.302708332089,292.988583490457,288.191388571794,286.113970767020,285.309041994516,284.733243126823,284.189019193475,282.574319206257,284.120379109830,287.795568057980,288.179078375760,290.209859138972,293.679673638155,297.453431448410,300.726288347892;0,288.700928736811,278.551672830084,273.400833959319,270.536547804349,267.833435583205,267.119414364878,265.972950018046,266.740920363958,268.048224971445,270.838385340352,270.778373480454,272.970259132319,275.506872347887,278.720407834140,281.813869092965;0,284.845821006168,269.394829178651,263.982926589081,260.478586413209,257.028965789929,255.931084916756,255.874470882376,256.430426703396,258.420242919460,257.808327020541,258.950655075076,261.079050323518,263.461085730423,266.382312892390,269.295763051135;0,288.386442360439,264.344752526028,257.213462364171,254.168296127581,250.527881300837,249.049345022729,250.073316495023,249.665324624047,248.602086912424,249.355944667699,250.714426186754,252.515083416491,254.990022645247,258.139224389126,258.885869213310;0,288.386442360439,267.197275532715,251.193959608514,247.553061326459,246.301141111655,244.695607301207,242.621990784403,242.304630618562,242.866111727694,243.758994026591,244.970247326866,246.821991594926,249.775586923996,251.245282116681,253.478417008787;0,288.386442360439,277.668290802935,252.854894387889,243.851167532952,241.861572413297,238.689990387976,238.067198500515,238.072941982365,238.685701547209,239.312989651019,240.673403883432,242.669277941474,245.301951037108,246.789302536782,247.789414843363;0,288.386442360439,277.504945286633,270.702819258252,245.731480615597,238.395305310031,236.119281963407,235.324944828075,235.181758472016,235.883544820460,236.679744588380,237.758701429304,239.923633193373,242.123394230695,242.998011528535,244.273734537053;0,288.386442360439,277.504945286633,279.349376222353,263.180462634460,241.569205761561,235.781254475789,234.445285156959,234.881842747232,234.822376790859,235.794452729420,237.439515459863,239.439460896780,241.356663529347,242.334213324245,244.486434215002;0,288.386442360439,277.504945286633,279.349376222353,299.505188255346,260.338046997911,239.404205178550,235.256510952508,234.880694514868,234.315938043290,236.319225658558,237.102712721133,239.012709272806,240.757763551380,241.336977805019,256.331160738088;0,288.386442360439,277.504945286633,279.349376222353,299.505188255346,320.026630425816,342.928313037200,241.524523052430,328.315966517739,244.549289572305,251.858270967766,240.732881082116,242.073820197020,244.535478307747,249.496579565711,263.930188372987;0,288.386442360439,277.504945286633,279.349376222353,299.505188255346,320.026630425816,342.928313037200,345.883623776508,328.315966517739,317.337354078743,314.624789096503,254.725548546873,250.384805432702,271.371327381584,265.474840242786,277.521724347837;0,288.386442360439,277.504945286633,279.349376222353,299.505188255346,320.026630425816,342.928313037200,345.883623776508,328.315966517739,319.749039003082,318.879022253509,311.782458169383,312.350604651759,319.747883103035,320.841917879101,308.256263223954],[0,0,0,0,0,0,0,0,0,0,0,0,0,0,0,0;0,514.035834811904,472.420001567292,468.560027988283,467.251130800260 ...(+7674 chars)])  Name6=EO HC  f_hc=f_hc  f_hc_3d=cat(3,[0,0,0,0,0,0,0,0,0,0,0,0,0,0,0,0;0,1.17332164513048e-05,9.91944779838112e-06,1.18397431832874e-05,1.41261124517862e-05,1.68353750922819e-05,1.92230735882396e-05,2.12492719202744e-05,2.26655444378036e-05,2.56418771066703e-05,2.91513785173347e-05,6.08912080367823e-05,6.92810181099260e-05,7.99093114577969e-05,8.16682563206722e-05,8.43028062960178e-05;0,7.47225604727487e-06,9.00571470212247e-06,1.12679775104734e-05,1.36908325704281e-05,1.60129853971162e-05,1.84116354582271e-05,2.05517089249360e-05,2.20830265583196e-05,2.47374328082615e-05,2.79253238491864e-05,6.55374159844044e-05,7.06533777289579e-05,8.00680789723272e-05,8.20564917047730e-05,8.43176890891716e-05;0,7.12638724691767e-06,9.18751596979668e-06,1.17486103156763e-05,1.41291038789512e-05,1.63503547064632e-05,1.89284579906511e-05,2.13132761100034e-05,2.52774728365996e-05,2.78197001590303e-05,3.04737469948358e-05,6.59703678640532e-05,7.14752781796029e-05,8.04572413784436e-05,8.21431368565846e-05,8.43158379056020e-05;0,7.08740753833251e-06,9.45860076094685e-06,1.24159627145423e-05,1.48377808638982e-05,1.75536071730362e-05,2.10835732172505e-05,2.43857604458034e-05,2.81344002484276e-05,3.16712984760753e-05,3.54149317512336e-05,6.70234643238439e-05,7.18030703850835e-05,8.04025094571605e-05,8.21521864399187e-05,8.43158379056020e-05;0,6.42029784391278e-06,9.30423013850866e-06,1.24594670913540e-05,1.58754153912287e-05,2.01360879812222e-05,2.39894781194505e-05,2.78116991470534e-05,3.20091516113821e-05,3.66658926338619e-05,4.02522787015150e-05,6.73163443175008e-05,7.19916146006501e-05,8.04376601529962e-05,8.21521864399187e-05,8.43158379056020e-05;0,8.10962672026543e-06,1.12314439478869e-05,1.46254832670078e-05,1.86960065261970e-05,2.32072093805049e-05,2.70580578738499e-05,3.19326549352392e-05,3.68906153692909e-05,4.11355936288291e-05,4.43439531716209e-05,6.74328888378119e-05,7.20298320403085e-05,8.04376666940561e-05,8.21521864399187e-05,8.43158379056020e-05;0,9.70568305659636e-06,1.35524796269905e-05,1.74907303306635e-05,2.23195050528327e-05,2.71644548563414e-05,3.19775889267411e-05,3.82925336531079e-05,4.08369896378773e-05,4.41028819611736e-05,4.80054038863669e-05,6.74471012961350e-05,7.20298414718821e-05,8.04376666940561e-05,8.21521864399187e-05,8.43158379056020e-05;0,9.63865029142607e-06,1.46918079771910e-05,2.04595547105073e-05,2.69774983732809e-05,3.18085523211663e-05,3.63396369925493e-05,4.08265095503008e-05,4.52038471281119e-05,5.76845232235684e-05,6.28551103306094e-05,6.74471012961350e-05,7.20298414718821e-05,8.04376666940561e-05,8.21521864399187e-05,8.43158379056020e-05;0,9.65039366574102e-06,1.66417340647553e-05,2.26472319605352e-05,2.85164261584315e-05,3.51031473211710e-05,4.03529865430686e-05,4.51863957190284e-05,5.24987255390409e-05,5.77133673662756e-05,6.28343383726769e-05,6.74471012961350e-05,7.20298414718821e-05,8.04376666940561e-05,8.21521864399187e-05,8.43158379056020e-05;0,9.65118996105956e-06,1.71412896644339e-05,2.60492310074593e-05,3.12466579051843e-05,3.72086432141992e-05,4.23460364695326e-05,4.66978128745530e-05,5.26941365537830e-05,5.77082025130950e-05,6.28810629252763e-05,6.74795758117571e-05,7.20298414718821e-05,8.04376666940561e-05,8.24455835847108e-05,8.50482683556549e-05;0,9.65093510615162e-06,1.72676140176090e-05,2.76722671320878e-05,3.51016413533288e-05,4.02998076525412e-05,4.62335609004000e-05,5.11269631246927e-05,5.67192113535543e-05,6.12095516518681e-05,6.59908288983150e-05,7.04812241655405e-05,7.69143137680485e-05,8.17334792434719e-05,8.46269545937590e-05,8.70828013242976e-05;0,9.67574585286823e-06,1.72911443197452e-05,2.77354161333053e-05,4.17911625710144e-05,4.44399014614598e-05,5.02272237676495e-05,5.56144760609065e-05,6.24109783511735e-05,6.60566167145197e-05,7.24326578450316e-05,7.79349119730411e-05,8.08524232167673e-05,8.41371713463231e-05,8.74935689244529e-05,8.95277600878926e-05;0,9.67482582182009e-06,1.73081599992859e-05,2.77734385910482e-05,4.36282027049877e-05,5.59619798022420e-05,5.67199402776834e-05,6.04005122539792e-05 ...(+10380 chars)])  Name7=EO CO  f_co=f_co  f_co_3d=cat(3,[0,0,0,0,0,0,0,0,0,0,0,0,0,0,0,0;0,1.94070845135971e-07,2.67140854368996e-07,8.38188462784441e-07,2.01307301292033e-06,1.99183632986460e-06,2.46540937098698e-06,2.77329805662432e-06,5.24763800208189e-06,6.01878203092976e-06,8.87334525400130e-06,6.04729962611755e-05,7.38543398595638e-05,9.33283946325456e-05,0.000106601894120056,0.000120601042402098;0,5.19153764640016e-07,1.04460758376968e-06,1.55968441468040e-06,3.54986301115943e-06,3.21324349383704e-06,3.83745509005428e-06,4.43208754055957e-06,7.70694636879153e-06,1.06177241749776e-05,1.38398448379505e-05,6.11191244372009e-05,7.54523614191272e-05,9.46701418521297e-05,0.000108447430131957,0.000121517759011285;0,6.89066751057659e-07,1.71803853251418e-06,1.54339938951999e-06,5.90884432444587e-06,3.65594096228512e-06,5.83168847010508e-06,8.40491738188118e-06,1.30859595119619e-05,1.59457490917740e-05,1.67713552202317e-05,6.33790689284524e-05,7.74726895841144e-05,9.71909530889313e-05,0.000109142230092030,0.000121625289064234;0,8.07527179959910e-07,1.28268140626446e-06,1.76576150812891e-06,2.43609026516920e-06,3.56896478462661e-06,5.38292800541256e-06,9.54860096466271e-06,1.30993903740458e-05,1.66019188532528e-05,2.19837470295026e-05,6.48629326947571e-05,7.88553089874429e-05,9.81187840412159e-05,0.000109473025132095,0.000121625289064234;0,1.05302438569732e-06,1.39819874620058e-06,1.96149907824741e-06,2.69769674745117e-06,4.06554733461386e-06,7.22491140250847e-06,1.07917039171025e-05,1.60427452046974e-05,2.22799188144221e-05,3.03731108008814e-05,6.57233226114596e-05,7.98458839825854e-05,9.84650857638634e-05,0.000109473017010648,0.000121625289064234;0,1.21878601061452e-05,1.89674754618221e-06,3.99180380773801e-06,7.45707310246567e-06,1.31550545718127e-05,1.74768201929713e-05,1.58125726273396e-05,1.50666198746385e-05,2.17299093329815e-05,2.97651400442293e-05,6.67660609164734e-05,8.06260603324165e-05,9.82957028494783e-05,0.000109473017010648,0.000121625289064234;0,1.01471389357925e-06,1.08478905999950e-05,9.46478487981287e-06,8.14982373703722e-06,1.77621696805127e-05,2.97175464378334e-05,3.88214498301098e-05,5.56610549463701e-05,7.20460477557571e-05,9.70866417398262e-05,6.69533890427884e-05,8.06429085525641e-05,9.82957028494783e-05,0.000109473017010648,0.000121625289064234;0,8.83157930515676e-07,4.04132275170136e-06,1.13018433486663e-05,3.72894648791464e-05,9.47260983821623e-06,1.18392027362989e-05,1.75967040913613e-05,2.62242669038525e-05,4.15272266453007e-05,5.29701284119496e-05,6.69448831512355e-05,8.06429085525641e-05,9.82957028494783e-05,0.000109473017010648,0.000121625289064234;0,1.01793974659128e-06,1.12612002657913e-05,7.17287220292544e-06,2.59169511913917e-05,8.17715620219110e-06,1.35977305201390e-05,2.25748025186746e-05,2.79142169053802e-05,4.12117086885715e-05,5.28406298953331e-05,6.69448831512355e-05,8.06429085525641e-05,9.82957028494783e-05,0.000109473017010648,0.000121625289064234;0,1.02572470118186e-06,1.12574609272404e-05,1.76775610547594e-05,1.66902308295477e-05,9.80163101741122e-06,1.42982242502242e-05,2.25156599359142e-05,2.79292050642812e-05,4.12425218296612e-05,5.28736882454880e-05,6.69448831512355e-05,8.06429085525641e-05,9.82957028494783e-05,0.000109473017010648,0.000121625289064234;0,1.02563870467461e-06,1.05794323336415e-05,3.20825049546582e-05,2.26736759500585e-05,1.55059993720495e-05,1.87497465692456e-05,2.81206510501001e-05,3.13806966913215e-05,4.49852495370279e-05,5.73280318362427e-05,6.76483934564418e-05,8.22881241846537e-05,0.000102442008339560,0.000119479223851685,0.000131447847813310;0,1.05024185279591e-06,1.04248095329839e-05,3.60112094977505e-05,0.000489320785952522,2.63998443472514e-05,4.32676977419324e-05,3.18628362145717e-05,0.000129355341590890,9.95373745870218e-05,0.000156336613045176,9.13327501489294e-05,0.000106777312459058,0.000118460138811775,0.000132300392986454,0.000152585093565902;0,1.05173101387095e-06,1.00675010018045e-05,3.60612957522358e-05,0.000613837437971602,0.000608304397430118,0.000314519090737616,4.28398768679800e-05 ...(+10344 chars)])  Name8=EO NOx  f_nox=f_nox  f_nox_3d=cat(3,[0,0,0,0,0,0,0,0,0,0,0,0,0,0,0,0;0,8.75024476827155e-08,4.15414639432748e-07,8.71073205780973e-07,1.39643333946097e-06,1.88338797087858e-06,2.81322491670027e-06,4.19936992423326e-06,5.67196743233119e-06,6.11901104678192e-06,6.35660152260592e-06,0.000109349783425841,0.000120982203220140,0.000152444535433487,0.000141607699560874,0.000136631353147245;0,3.79429540411136e-07,1.31234931125769e-06,2.59523910658250e-06,4.03219005106766e-06,5.83740067662685e-06,7.88061607973418e-06,1.02403254940097e-05,1.33614022021932e-05,1.46616823513197e-05,1.55633098842551e-05,0.000113651910664498,0.000134143305878514,0.000153547344744979,0.000142010254921491,0.000137223103230791;0,7.61380615375592e-07,2.42563446421634e-06,4.29836145491423e-06,7.05819841710222e-06,1.11665365742608e-05,1.49350971302275e-05,1.70302662643071e-05,1.89239000507646e-05,2.11519897895623e-05,2.89731994558040e-05,0.000124892193947227,0.000140610812895066,0.000154048191780538,0.000142389121090470,0.000137417029454528;0,1.30616517341511e-06,3.55100147815598e-06,5.80789909952846e-06,1.01523393815916e-05,1.65852513891373e-05,2.20139245805219e-05,2.12491121174890e-05,1.97534549564683e-05,2.55852703400335e-05,4.50749634155717e-05,0.000127244665510254,0.000143204645839380,0.000154325349885329,0.000142406264585723,0.000137417029454528;0,3.35457160907255e-06,6.09785244195068e-06,8.17508166664579e-06,1.11615326646696e-05,1.46473073753065e-05,2.08231605399363e-05,2.37035595754022e-05,2.77511981066398e-05,4.54802557161102e-05,6.62093829449065e-05,0.000128872440293165,0.000145003063859556,0.000154589177969718,0.000142406244686937,0.000137417029454528;0,5.80007395024816e-06,1.10625995224393e-05,1.56488776930843e-05,1.69424416192163e-05,1.63638262690047e-05,2.27014031730039e-05,3.45061890076058e-05,4.67329454059615e-05,7.18353048726039e-05,7.93190928733020e-05,0.000129919835796284,0.000145380426940981,0.000154600992707205,0.000142406244686937,0.000137417029454528;0,1.20802213200447e-05,1.64899812177677e-05,2.54589826833969e-05,3.05538655205608e-05,2.75794681889144e-05,3.51199489702964e-05,6.10379039522278e-05,7.06186320720783e-05,7.51716765155704e-05,7.60676006641496e-05,0.000130158762389046,0.000145375598916073,0.000154600992707205,0.000142406244686937,0.000137417029454528;0,1.18050945523770e-05,1.91780235835761e-05,3.14118176317666e-05,4.32392665373654e-05,5.55321768277827e-05,6.93582908700481e-05,8.00356397081443e-05,8.88879541399358e-05,0.000111035845175980,0.000119234071791238,0.000130161059819193,0.000145375598916073,0.000154600992707205,0.000142406244686937,0.000137417029454528;0,1.15521976623953e-05,1.88888954954831e-05,3.03480007064977e-05,4.52801810896987e-05,6.24498622347551e-05,7.90347353560890e-05,9.38065652089259e-05,0.000106040931199075,0.000111210999379892,0.000119305839042719,0.000130161059819193,0.000145375598916073,0.000154600992707205,0.000142406244686937,0.000137417029454528;0,1.15447503706373e-05,1.99534696973802e-05,3.04555139869586e-05,4.49832303985015e-05,6.25400954728056e-05,7.92948516913183e-05,9.37945571843342e-05,0.000106031507125979,0.000111234433862100,0.000119264450507825,0.000130161059819193,0.000145375598916073,0.000154600992707205,0.000142406244686937,0.000137417029454528;0,1.15438751719152e-05,2.02363112720891e-05,3.17354192155619e-05,4.44238353891855e-05,6.22684149281069e-05,8.01493783520780e-05,9.66624784954232e-05,0.000107242607010646,0.000114322972698626,0.000122011205152926,0.000133937207061123,0.000146190016679633,0.000152798731866827,0.000140401028078364,0.000136000910706728;0,1.16815863626166e-05,2.03856875570182e-05,3.21694024637262e-05,2.80888593696816e-05,6.07461384329539e-05,7.74762309696713e-05,9.56402387295794e-05,0.000102846717298022,0.000115578123240838,0.000124460354013458,0.000144100860173105,0.000148175433614933,0.000148645337564915,0.000141054413692415,0.000134268997080035;0,1.16815065370073e-05,2.04558501042666e-05,3.22263512496322e-05,2.83143643584321e-05,3.72924154277625e-05,6.36302622776627e-05,9.68204466904155e-05 ...(+10380 chars)])  Name9=EO CO2  f_co2=f_co2  f_co2_3d=cat(3,[0,0,0,0,0,0,0,0,0,0,0,0,0,0,0,0;0,0.000515045852007081,0.000680311906512726,0.000870603209158873,0.00105157911357196,0.00123759294298862,0.00142061554632062,0.00161342000193231,0.00178579000250817,0.00194081343961215,0.00209692926540666,0.00747459043422927,0.00797741972685754,0.00932956329515088,0.00926654375950917,0.00941580473571887;0,0.000676283242522166,0.000921696147404133,0.00117294979125748,0.00141079642682370,0.00164764543141983,0.00188617276314695,0.00213755931535274,0.00235470405452953,0.00257134518761704,0.00278394395484521,0.00772348560939706,0.00875491874023005,0.00942656064430304,0.00931382737645156,0.00942851883695287;0,0.000844140993791010,0.00115944257641566,0.00146434927490643,0.00175620721781783,0.00206369489148816,0.00236806317445392,0.00267238828927539,0.00294762560448119,0.00321090254711249,0.00347662913384927,0.00853011211377682,0.00906284283641105,0.00951542804480680,0.00933427150528462,0.00943036429087221;0,0.00102414423888895,0.00139151691633023,0.00175638320378358,0.00213194953128991,0.00250638339531224,0.00286176340622650,0.00320922349270804,0.00352245133354472,0.00385519677354598,0.00420942467438452,0.00865425395011219,0.00912889172651981,0.00953931229247772,0.00933803303486770,0.00943036429087221;0,0.00119587441683547,0.00162823412341072,0.00206263642284447,0.00249798186087907,0.00291175764295492,0.00332201228730209,0.00371454324022988,0.00409749227637894,0.00452609942728713,0.00492978645576279,0.00870429060871990,0.00917043364477652,0.00954511880932982,0.00933803158081780,0.00943036429087221;0,0.00126643488829815,0.00186888897813569,0.00235979635755733,0.00284031799131893,0.00327375940140541,0.00371556391579781,0.00417072618441846,0.00464518163541044,0.00510019834242980,0.00548230063895929,0.00873530585053485,0.00918277732132748,0.00954597668059092,0.00933803158081780,0.00943036429087221;0,0.00164262319497678,0.00211982435438154,0.00264338113246542,0.00320325215606864,0.00366324851282020,0.00411200348060070,0.00458075659018702,0.00494175476299997,0.00526929500276456,0.00548167147080596,0.00874168498536456,0.00918334809647699,0.00954597668059092,0.00933803158081780,0.00943036429087221;0,0.00166597433853797,0.00236116698911612,0.00299285841534142,0.00357970735725608,0.00424464507882457,0.00479116972118136,0.00531572273939085,0.00584295300424232,0.00767656186949225,0.00824085073499353,0.00874191334023930,0.00918334809647699,0.00954597668059092,0.00933803158081780,0.00943036429087221;0,0.00167128931685933,0.00263900459237861,0.00327907924733082,0.00392535499251438,0.00477846006149459,0.00552935227067135,0.00620887927415138,0.00705444206032986,0.00768752907360983,0.00824450776516289,0.00874191334023930,0.00918334809647699,0.00954597668059092,0.00933803158081780,0.00943036429087221;0,0.00167139363161070,0.00274623797705486,0.00375219796269222,0.00431625814871545,0.00496672394448067,0.00561736915056791,0.00621258578074294,0.00705454451290115,0.00768816378153152,0.00824514385878778,0.00874191334023930,0.00918334809647699,0.00954597668059092,0.00933803158081780,0.00943036429087221;0,0.00167138030544215,0.00276417790567446,0.00410111244134831,0.00481040538402329,0.00541243502753216,0.00606933849929676,0.00669575318459739,0.00736430724839299,0.00794407764006462,0.00844026324558207,0.00889797219552370,0.00925460885760685,0.00957679897802262,0.00954299867762758,0.00959172739745095;0,0.00167653452929439,0.00277255055448440,0.00414715928538353,0.00511002445032008,0.00593438092758995,0.00655354350555542,0.00723091507059225,0.00787448438274641,0.00840977181936236,0.00892408486953961,0.00943229831882970,0.00971900535178170,0.00989237898139211,0.00988486514858594,0.00984879798820839;0,0.00167652376041293,0.00277707206678690,0.00415146404665018,0.00545456773358663,0.00623247381735294,0.00688936293874938,0.00777088867047902,0.00806663077390940,0.00872764319765997,0.00916247219222665,0.00988838385054398,0.0101214558077607,0.0102188435073538,0.0102465020325985,0.0100170041167877;0,0.00167629597087569 ...(+9684 chars)])  Name10=Brake Torque  f_pm=f_pm  f_pm_3d=cat(3,[0,0,0,0,0,0,0,0,0,0,0,0,0,0,0,0;0,0,0,0,0,0,0,0,0,0,0,0,0,0,0,0;0,0,0,0,0,0,0,0,0,0,0,0,0,0,0,0;0,0,0,0,0,0,0,0,0,0,0,0,0,0,0,0;0,0,0,0,0,0,0,0,0,0,0,0,0,0,0,0;0,0,0,0,0,0,0,0,0,0,0,0,0,0,0,0;0,0,0,0,0,0,0,0,0,0,0,0,0,0,0,0;0,0,0,0,0,0,0,0,0,0,0,0,0,0,0,0;0,0,0,0,0,0,0,0,0,0,0,0,0,0,0,0;0,0,0,0,0,0,0,0,0,0,0,0,0,0,0,0;0,0,0,0,0,0,0,0,0,0,0,0,0,0,0,0;0,0,0,0,0,0,0,0,0,0,0,0,0,0,0,0;0,0,0,0,0,0,0,0,0,0,0,0,0,0,0,0;0,0,0,0,0,0,0,0,0,0,0,0,0,0,0,0;0,0,0,0,0,0,0,0,0,0,0,0,0,0,0,0;0,0,0,0,0,0,0,0,0,0,0,0,0,0,0,0],[0,0,0,0,0,0,0,0,0,0,0,0,0,0,0,0;0,0,0,0,0,0,0,0,0,0,0,0,0,0,0,0;0,0,0,0,0,0,0,0,0,0,0,0,0,0,0,0;0,0,0,0,0,0,0,0,0,0,0,0,0,0,0,0;0,0,0,0,0,0,0,0,0,0,0,0,0,0,0,0;0,0,0,0,0,0,0,0,0,0,0,0,0,0,0,0;0,0,0,0,0,0,0,0,0,0,0,0,0,0,0,0;0,0,0,0,0,0,0,0,0,0,0,0,0,0,0,0;0,0,0,0,0,0,0,0,0,0,0,0,0,0,0,0;0,0,0,0,0,0,0,0,0,0,0,0,0,0,0,0;0,0,0,0,0,0,0,0,0,0,0,0,0,0,0,0;0,0,0,0,0,0,0,0,0,0,0,0,0,0,0,0;0,0,0,0,0,0,0,0,0,0,0,0,0,0,0,0;0,0,0,0,0,0,0,0,0,0,0,0,0,0,0,0;0,0,0,0,0,0,0,0,0,0,0,0,0,0,0,0;0,0,0,0,0,0,0,0,0,0,0,0,0,0,0,0],[0,0,0,0,0,0,0,0,0,0,0,0,0,0,0,0;0,0,0,0,0,0,0,0,0,0,0,0,0,0,0,0;0,0,0,0,0,0,0,0,0,0,0,0,0,0,0,0;0,0,0,0,0,0,0,0,0,0,0,0,0,0,0,0;0,0,0,0,0,0,0,0,0,0,0,0,0,0,0,0;0,0,0,0,0,0,0,0,0,0,0,0,0,0,0,0;0,0,0,0,0,0,0,0,0,0,0,0,0,0,0,0;0,0,0,0,0,0,0,0,0,0,0,0,0,0,0,0;0,0,0,0,0,0,0,0,0,0,0,0,0,0,0,0;0,0,0,0,0,0,0,0,0,0,0,0,0,0,0,0;0,0,0,0,0,0,0,0,0,0,0,0,0,0,0,0;0,0,0,0,0,0,0,0,0,0,0,0,0,0,0,0;0,0,0,0,0,0,0,0,0,0,0,0,0,0,0,0;0,0,0,0,0,0,0,0,0,0,0,0,0,0,0,0;0,0,0,0,0,0,0,0,0,0,0,0,0,0,0,0;0,0,0,0,0,0,0,0,0,0,0,0,0,0,0,0])  aMode=1  CalMapsData={'', '', 'MappedEngine-Nonfiring', 'MappedEngine-Torque'}
      settings: LibrarySourceBlock=autolibenginesystems/Mapped SI Engine
  Mux : Mux  Inputs=1
  Product : Product
  Product1 : Product  Inputs=*/
  Product2 : Product
  Terminator{,1..2,4,12..13} (6 alike) : Terminator
  Three-Way Catalyst : Subsystem
  div0protect - poly1 : autolibutils/div0protect - poly  thresh=0.01  ZeroCross1=off  aMode=aMode
  EngTrq : Outport  Unit=N*m  VectorParamsAs1DForOutWhenUnconnected=off
  EngSpdOut : Outport  Port=2  VectorParamsAs1DForOutWhenUnconnected=off
  Map : Outport  Port=3  Unit=Pa  VectorParamsAs1DForOutWhenUnconnected=off
  Mat : Outport  Port=4  Unit=K  VectorParamsAs1DForOutWhenUnconnected=off
  ThrPosPct : Outport  Port=5  VectorParamsAs1DForOutWhenUnconnected=off
  WgAreaPct : Outport  Port=6  VectorParamsAs1DForOutWhenUnconnected=off
  IntkCamPhase : Outport  Port=7  VectorParamsAs1DForOutWhenUnconnected=off
  ExhCamPhase : Outport  Port=8  VectorParamsAs1DForOutWhenUnconnected=off
  TurboRackPos : Outport  Port=9  VectorParamsAs1DForOutWhenUnconnected=off
  EgrVlvAreaPct : Outport  Port=10  VectorParamsAs1DForOutWhenUnconnected=off
  VarCompRatioPos : Outport  Port=11  VectorParamsAs1DForOutWhenUnconnected=off
  IntkVlvLift : Outport  Port=12  VectorParamsAs1DForOutWhenUnconnected=off
  VarIntkRunLen : Outport  Port=13  VectorParamsAs1DForOutWhenUnconnected=off
  IntkSwirlVlvPos : Outport  Port=14  VectorParamsAs1DForOutWhenUnconnected=off
  FuelFlw : Outport  Port=15  Unit=kg/s  VectorParamsAs1DForOutWhenUnconnected=off
  FuelVolFlw : Outport  Port=16  Unit=m^3/s  VectorParamsAs1DForOutWhenUnconnected=off
  IntkPortFlw : Outport  Port=17  VectorParamsAs1DForOutWhenUnconnected=off
  NormAirChrg : Outport  Port=18  VectorParamsAs1DForOutWhenUnconnected=off
  ExhManGasTemp : Outport  Port=19  VectorParamsAs1DForOutWhenUnconnected=off
  Afr : Outport  Port=20  Unit=1  VectorParamsAs1DForOutWhenUnconnected=off
  TurboSpd : Outport  Port=21  Unit=rad/s  VectorParamsAs1DForOutWhenUnconnected=off
  TurbPrsRatio : Outport  Port=22  Unit=1  VectorParamsAs1DForOutWhenUnconnected=off
  CompPrsRatio : Outport  Port=23  Unit=1  VectorParamsAs1DForOutWhenUnconnected=off
  TurbTempOut : Outport  Port=24  Unit=K  VectorParamsAs1DForOutWhenUnconnected=off
  CompTempOut : Outport  Port=25  Unit=K  VectorParamsAs1DForOutWhenUnconnected=off
  EgrPct : Outport  Port=26  Unit=%  VectorParamsAs1DForOutWhenUnconnected=off
  EgrMassFlwRate : Outport  Port=27  Unit=kg/s  VectorParamsAs1DForOutWhenUnconnected=off
  EgrCoolerTempOut : Outport  Port=28  Unit=K  VectorParamsAs1DForOutWhenUnconnected=off
  IntercoolerTempOut : Outport  Port=29  Unit=K  VectorParamsAs1DForOutWhenUnconnected=off
  BSFC : Outport  Port=30  VectorParamsAs1DForOutWhenUnconnected=off
  TP HC : Outport  Port=31  VectorParamsAs1DForOutWhenUnconnected=off
  TP CO : Outport  Port=32  VectorParamsAs1DForOutWhenUnconnected=off
  TP NOx : Outport  Port=33  VectorParamsAs1DForOutWhenUnconnected=off
  TP CO2 : Outport  Port=34  VectorParamsAs1DForOutWhenUnconnected=off
  Iat : Outport  Port=35  Unit=K  VectorParamsAs1DForOutWhenUnconnected=off
  Ect : Outport  Port=36  Unit=K  VectorParamsAs1DForOutWhenUnconnected=off
  EgrVlvDeltaPrs : Outport  Port=37  Unit=Pa  VectorParamsAs1DForOutWhenUnconnected=off
  EgrVlvInTemp : Outport  Port=38  Unit=K  VectorParamsAs1DForOutWhenUnconnected=off
  CylPrs : Outport  Port=39  VectorParamsAs1DForOutWhenUnconnected=off
  EngTrqCrk : Outport  Port=40  VectorParamsAs1DForOutWhenUnconnected=off
  CrkAng : Outport  Port=41  VectorParamsAs1DForOutWhenUnconnected=off
  wires:
  Mapped SI Engine/1 -> Bus Selector/1
  Bus Selector/6 -> ExhManGasTemp/1, Three-Way Catalyst/1(Exhaust Temperature)  "<ExhManGasTemp>"
  Product1/1 -> Afr/1, Three-Way Catalyst/2(Afr)
  EngSpd/1 -> Accessory Load Model/2(EngSpd), Mapped SI Engine/2
  Bus Selector/1 -> EngSpdOut/1  "<EngSpd>"
  Bus Selector/2 -> Product/1  "<FuelMassFlw>"
  Bus Selector/4 -> IntkPortFlw/1  "<IntkGasMassFlw>"
  Bus Selector/9 -> Three-Way Catalyst/3(EO HC)  "<EoHC>"
  Bus Selector/10 -> Three-Way Catalyst/4(EO CO)  "<EoCO>"
  Bus Selector/11 -> Three-Way Catalyst/5(EO NOx)  "<EoNOx>"
  Bus Selector/12 -> Mux/1  "<EoCO2>"
  Three-Way Catalyst/1(TP HC) -> TP HC/1
  Three-Way Catalyst/2(TP CO) -> TP CO/1
  Three-Way Catalyst/3(TP NOx) -> TP NOx/1
  Mux/1 -> TP CO2/1
  TrqCmd/1 -> Electronic Throttle Actuator Dynamics/1
  Bus Selector/8 -> BSFC/1  "<Bsfc>"
  Bus Selector/5 -> NormAirChrg/1  "<NrmlzdAirChrg>"
  Electronic Throttle Actuator Dynamics/1 -> Mapped SI Engine/1
  IntkCamPhaseCmd/1 -> Actuators/6(IntkCamPhaseCmd)
  Ground16/1 -> EgrCoolerTempOut/1
  Ground14/1 -> EgrPct/1
  Ground13/1 -> IntercoolerTempOut/1
  Ground12/1 -> CompTempOut/1
  FuelMainSoi/1 -> Actuators/4(FuelMainSoiCmd)
  EgrVlvAreaPctCmd/1 -> Actuators/9(EgrVlvAreaPctCmd)
  Ground11/1 -> TurbTempOut/1
  ExhCamPhaseCmd/1 -> Actuators/7(ExhCamPhaseCmd)
  Ground9/1 -> TurbPrsRatio/1
  Ground8/1 -> TurboSpd/1
  SpkAdv/1 -> Actuators/5(SpkAdvCmd)
  AmbTemp/1 -> Terminator12/1
  Ground15/1 -> EgrMassFlwRate/1
  TurboRackPosCmd/1 -> Actuators/8(TurboRackPosCmd)
  ThrPosPctCmd/1 -> Actuators/1(ThrPosPctCmd)
  WgAreaPctCmd/1 -> Actuators/2(WgAreaPctCmd)
  InjPw/1 -> Actuators/3(InjPwCmd)
  Ground10/1 -> CompPrsRatio/1
  Ground1/1 -> Mat/1
  Ground/1 -> Map/1
  AmbPrs/1 -> Terminator13/1
  IntkVlvLiftCmd/1 -> Actuators/11(IntkVlvLiftCmd)
  VarCompRatioPosCmd/1 -> Actuators/10(VarCompRatioPosCmd)
  VarIntkRunLenCmd/1 -> Actuators/12(VarIntkRunLenCmd)
  IntkSwirlVlvPosCmd/1 -> Actuators/13(IntkSwirlVlvPosCmd)
  UndHdFlwVel/1 -> Terminator4/1
  Actuators/1(ThrPosPct) -> ThrPosPct/1
  Actuators/2(WgAreaPct) -> WgAreaPct/1
  Actuators/3(InjPw) -> Terminator1/1
  Actuators/4(SpkAdv) -> Terminator2/1
  Actuators/5(IntkCamPhase) -> IntkCamPhase/1
  Actuators/6(ExhCamPhase) -> ExhCamPhase/1
  Actuators/7(TurboRackPos) -> TurboRackPos/1
  Actuators/8(EgrVlvAreaPct) -> EgrVlvAreaPct/1
  Actuators/9(VarCompRatioPos) -> VarCompRatioPos/1
  Actuators/10(IntkVlvLift) -> IntkVlvLift/1
  Actuators/11(VarIntkRunLen) -> VarIntkRunLen/1
  Actuators/12(IntkSwirlVlvPos) -> IntkSwirlVlvPos/1
  Constant/1 -> Ect/1
  Ground2/1 -> EgrVlvInTemp/1
  Ground3/1 -> EgrVlvDeltaPrs/1
  Ground4/1 -> Iat/1
  Accessory Load Model/2(EngTrqOut) -> EngTrq/1
  Mapped SI Engine/2 -> Accessory Load Model/1(EngTrqIn)
  Accessory Load Model/1(PwrInfo) -> Terminator/1
  Bus Selector/3 -> Product2/1  "<FuelVolFlw>"
  Product/1 -> FuelFlw/1
  Bus Selector/7 -> Product1/1  "<Afr>"
  Product2/1 -> FuelVolFlw/1
  [ClsdLpFuelMult] -> div0protect - poly1/1
  ClsdLpFuelMult/1 -> [ClsdLpFuelMult]
  div0protect - poly1/1 -> Product1/2, Product2/2, Product/2
  Ground5/1 -> CylPrs/1
  Ground6/1 -> EngTrqCrk/1
  Ground7/1 -> CrkAng/1
